simulink model "Examples_Session_2"  (R2023b)
settings: Solver=VariableStepAuto  StartTime=0.0  StopTime=10.0  RelTol=1e-3
libraries: simulink x13
settings Model: Creator=hp  LastModifiedBy=hp

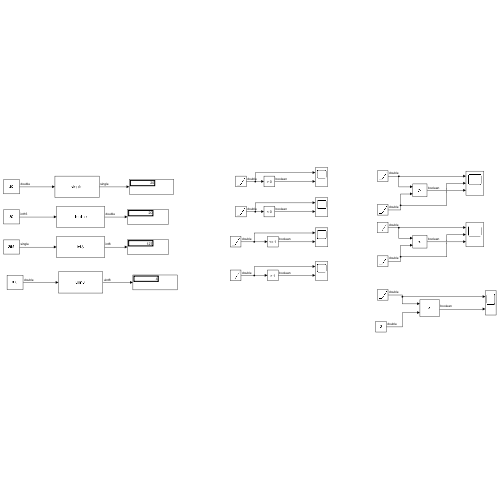
[thumbnail: Simulink's stored preview of the top-level diagram]
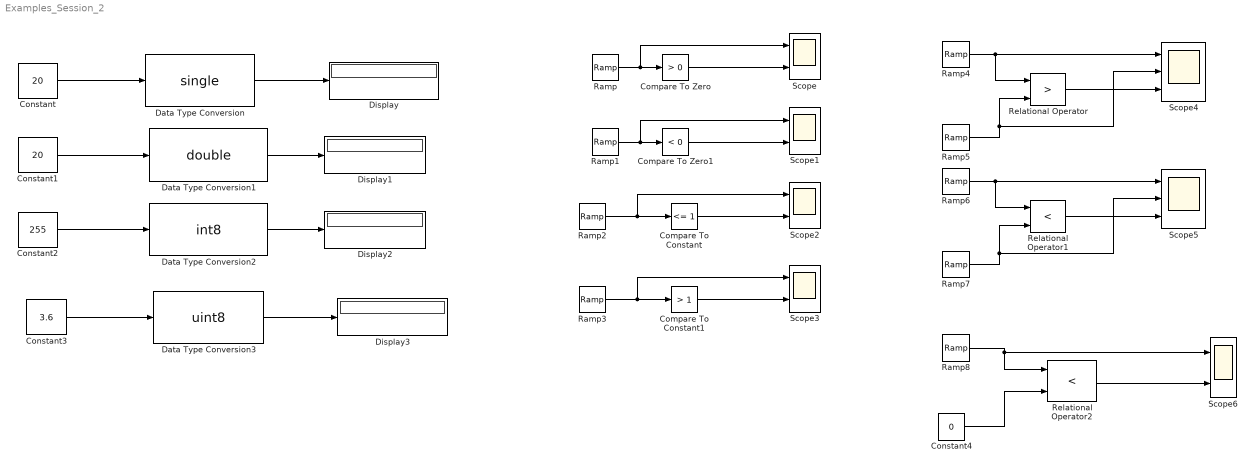
== system Examples_Session_2 ==
  Compare To Constant : simulink/Logic and Bit Operations/Compare To Constant  relop=<=  const=1  OutDataTypeStr=boolean
  Compare To Constant1 : simulink/Logic and Bit Operations/Compare To Constant  relop=>  const=1  OutDataTypeStr=boolean
  Compare To Zero : simulink/Logic and Bit Operations/Compare To Zero  relop=>  OutDataTypeStr=boolean
  Compare To Zero1 : simulink/Logic and Bit Operations/Compare To Zero  relop=<  OutDataTypeStr=boolean
  Constant : Constant  Value=20
  Constant1 : Constant  Value=20  OutDataTypeStr=int16
  Constant2 : Constant  Value=255  OutDataTypeStr=single
  Constant3 : Constant  Value=3.6
  Constant4 : Constant  Value=0
  Data Type Conversion : DataTypeConversion  OutDataTypeStr=single  SaturateOnIntegerOverflow=off  RndMeth=Floor
  Data Type Conversion1 : DataTypeConversion  OutDataTypeStr=double  SaturateOnIntegerOverflow=off  RndMeth=Floor
  Data Type Conversion2 : DataTypeConversion  OutDataTypeStr=int8  RndMeth=Floor
  Data Type Conversion3 : DataTypeConversion  OutDataTypeStr=uint8  RndMeth=Round  SaturateOnIntegerOverflow=off
  Display{,1..3} (4 alike) : Display
  Ramp : simulink/Sources/Ramp  slope=1  start=0  InitialOutput=-0.5
  Ramp1 : simulink/Sources/Ramp  slope=1  start=0  InitialOutput=-0.5
  Ramp2 : simulink/Sources/Ramp  slope=-0.5  start=0  InitialOutput=2
  Ramp3 : simulink/Sources/Ramp  slope=-0.5  start=0  InitialOutput=2
  Ramp4 : simulink/Sources/Ramp  slope=1  start=0  InitialOutput=-4
  Ramp5 : simulink/Sources/Ramp  slope=-1  start=0  InitialOutput=8
  Ramp6 : simulink/Sources/Ramp  slope=1  start=0  InitialOutput=-4
  Ramp7 : simulink/Sources/Ramp  slope=-1  start=0  InitialOutput=8
  Ramp8 : simulink/Sources/Ramp  slope=1  start=0  InitialOutput=-4
  Relational Operator : RelationalOperator  Operator=>  OutDataTypeStr=boolean  RndMeth=Simplest  InputSameDT=off
  Relational Operator1 : RelationalOperator  Operator=<  OutDataTypeStr=boolean  RndMeth=Simplest  InputSameDT=off
  Relational Operator2 : RelationalOperator  Operator=<  OutDataTypeStr=boolean  RndMeth=Simplest  InputSameDT=off
  Scope{,1..3,6} (5 alike) : Scope  NumInputPorts=2
  Scope4 : Scope  NumInputPorts=3
  Scope5 : Scope  NumInputPorts=3
  wires:
  Constant/1 -> Data Type Conversion/1
  Data Type Conversion/1 -> Display/1
  Constant1/1 -> Data Type Conversion1/1
  Data Type Conversion1/1 -> Display1/1
  Data Type Conversion2/1 -> Display2/1
  Constant2/1 -> Data Type Conversion2/1
  Data Type Conversion3/1 -> Display3/1
  Constant3/1 -> Data Type Conversion3/1
  Ramp/1 -> Scope/1, Compare To Zero/1
  Compare To Zero/1 -> Scope/2
  Compare To Zero1/1 -> Scope1/2
  Ramp1/1 -> Compare To Zero1/1, Scope1/1
  Ramp2/1 -> Scope2/1, Compare To Constant/1
  Compare To Constant/1 -> Scope2/2
  Compare To Constant1/1 -> Scope3/2
  Ramp3/1 -> Compare To Constant1/1, Scope3/1
  Ramp4/1 -> Scope4/1, Relational Operator/1
  Ramp5/1 -> Relational Operator/2, Scope4/2
  Relational Operator/1 -> Scope4/3
  Relational Operator1/1 -> Scope5/3
  Ramp7/1 -> Scope5/2, Relational Operator1/2
  Ramp6/1 -> Relational Operator1/1, Scope5/1
  Ramp8/1 -> Scope6/1, Relational Operator2/1
  Constant4/1 -> Relational Operator2/2
  Relational Operator2/1 -> Scope6/2
